simulink model "SineWaves"  (R2013a)
settings: Solver=ode45  StartTime=0.0  StopTime=1000  RelTol=1e-3
libraries: dspmtrx3 x7
settings Model: Creator=100432553  LastModifiedBy=Dolby
settings DataIOCC: SignalLoggingSaveFormat=ModelDataLogs
settings DebuggingCC: UnderspecifiedInitializationDetection=Simplified  MultiTaskDSMMsg=warning  MultiTaskCondExecSysMsg=none  StateNameClashWarn=none  StrictBusMsg=None
settings RTWCC: IncludeERTFirstTime=on
settings GRTTargetCC: CodeReplacementLibrary=None  CPPClassGenCompliant=on

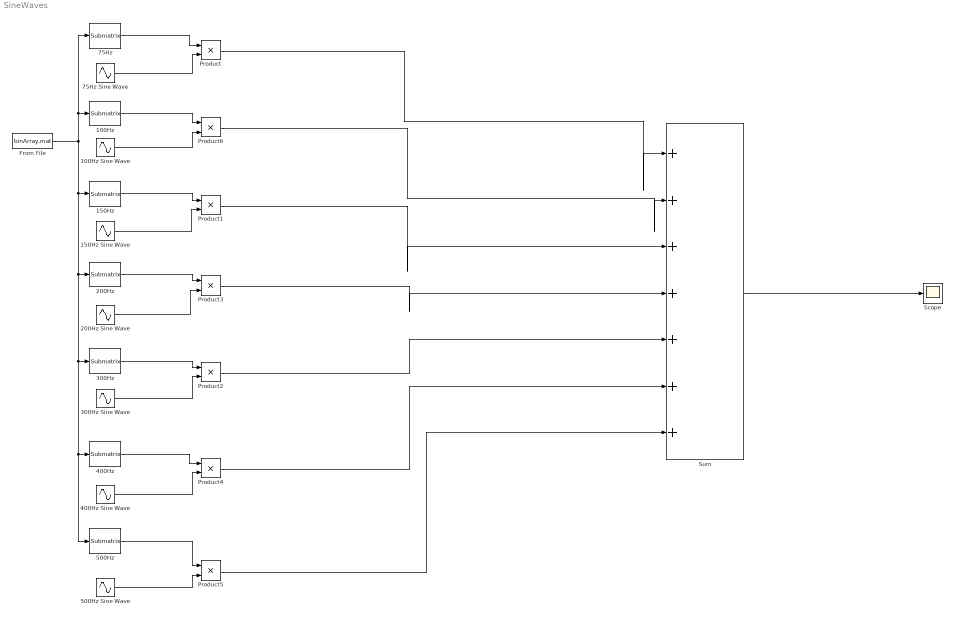
== system SineWaves ==
  100Hz : dspmtrx3/Submatrix  RowSpan=One row  RowStartMode=Index  RowStartIndex=2  RowEndMode=Last  RowEndIndex=1  ColSpan=Range of columns  ColStartMode=First  ColStartIndex=1  ColEndMode=Last  ColEndIndex=1
  100Hz Sine Wave : Sin  Amplitude=1 + rand()  Frequency=1.7453  SampleTime=1/8000
  150Hz : dspmtrx3/Submatrix  RowSpan=One row  RowStartMode=Index  RowStartIndex=3  RowEndMode=Last  RowEndIndex=1  ColSpan=Range of columns  ColStartMode=First  ColStartIndex=1  ColEndMode=Last  ColEndIndex=1
  150Hz Sine Wave : Sin  Amplitude=1 + rand()  Frequency=2.618  SampleTime=1/8000
  200Hz : dspmtrx3/Submatrix  RowSpan=One row  RowStartMode=Index  RowStartIndex=4  RowEndMode=Last  RowEndIndex=1  ColSpan=Range of columns  ColStartMode=First  ColStartIndex=1  ColEndMode=Last  ColEndIndex=1
  200Hz Sine Wave : Sin  Amplitude=1 + rand()  Frequency=3.4907  SampleTime=1/8000
  300Hz : dspmtrx3/Submatrix  RowSpan=One row  RowStartMode=Index  RowStartIndex=5  RowEndMode=Last  RowEndIndex=1  ColSpan=Range of columns  ColStartMode=First  ColStartIndex=1  ColEndMode=Last  ColEndIndex=1
  300Hz Sine Wave : Sin  Amplitude=1 + rand()  Frequency=5.236  SampleTime=1/8000
  400Hz : dspmtrx3/Submatrix  RowSpan=One row  RowStartMode=Index  RowStartIndex=6  RowEndMode=Last  RowEndIndex=1  ColSpan=Range of columns  ColStartMode=First  ColStartIndex=1  ColEndMode=Last  ColEndIndex=1
  400Hz Sine Wave : Sin  Amplitude=1 + rand()  Frequency=6.9813  SampleTime=1/8000
  500Hz : dspmtrx3/Submatrix  RowSpan=One row  RowStartMode=Last  RowStartIndex=1  RowEndMode=Last  RowEndIndex=1  ColSpan=Range of columns  ColStartMode=First  ColStartIndex=1  ColEndMode=Last  ColEndIndex=1
  500Hz Sine Wave : Sin  Amplitude=1 + rand()  Frequency=8.7266  SampleTime=1/8000
  75Hz : dspmtrx3/Submatrix  RowSpan=One row  RowStartMode=First  RowStartIndex=1  RowEndMode=Last  RowEndIndex=1  ColSpan=Range of columns  ColStartMode=First  ColStartIndex=1  ColEndMode=Last  ColEndIndex=1
  75Hz Sine Wave : Sin  Amplitude=1 + rand()  Frequency=1.309  SampleTime=1/8000
  From File : FromFile  FileName=binArray.mat  SampleTime=0  ExtrapolationBeforeFirstDataPoint=Ground value  InterpolationWithinTimeRange=Zero order hold  ExtrapolationAfterLastDataPoint=Ground value
  Product{,1..6} (7 alike) : Product
  Scope : Scope
  Sum : Sum  Inputs=|+++++++
  wires:
  From File/1 -> 100Hz/1, 75Hz/1, 150Hz/1, 500Hz/1, 400Hz/1, 300Hz/1, 200Hz/1
  150Hz/1 -> Product1/1
  150Hz Sine Wave/1 -> Product1/2
  200Hz Sine Wave/1 -> Product3/2
  200Hz/1 -> Product3/1
  100Hz Sine Wave/1 -> Product6/2
  100Hz/1 -> Product6/1
  300Hz Sine Wave/1 -> Product2/2
  300Hz/1 -> Product2/1
  75Hz/1 -> Product/1
  75Hz Sine Wave/1 -> Product/2
  400Hz/1 -> Product4/1
  400Hz Sine Wave/1 -> Product4/2
  500Hz/1 -> Product5/1
  500Hz Sine Wave/1 -> Product5/2
  Product/1 -> Sum/1
  Product6/1 -> Sum/2
  Product1/1 -> Sum/3
  Product3/1 -> Sum/4
  Product2/1 -> Sum/5
  Product4/1 -> Sum/6
  Product5/1 -> Sum/7
  Sum/1 -> Scope/1
